simulink model "UUV_model_sim"  (R2020a)
settings: Solver=VariableStepAuto  StartTime=0.0  StopTime=20  FixedStep=0.01  RelTol=1e-3
model workspace (MAT data in the model file):
  NED = [0; 0; 0; 0; 0; 0]
  NED_dot = [0; 0; 0; 0; 0; 0]
  a = [0; 0; 0; 0; 0; 0]
  vel = [0; 0; 0; 0; 0; 0]
libraries: simulink x2
settings Model: Creator=Sebas  LastModifiedBy=Sebas

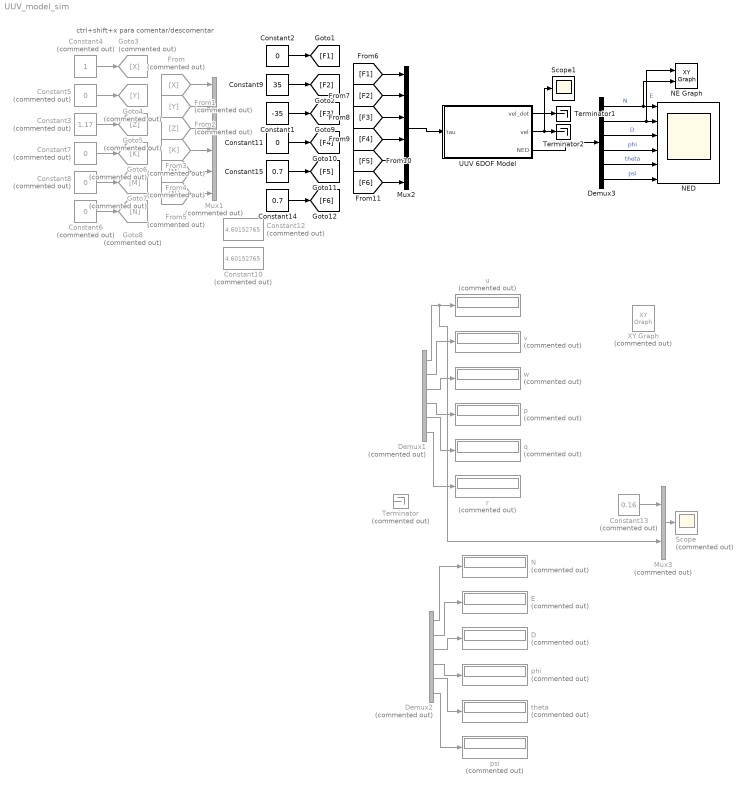
== system UUV_model_sim ==
  note: ctrl+shift+x para comentar/descomentar
  Constant1 : Constant  Value=-35
  Constant10 : Constant  Commented=on  Value=4.60152765
  Constant11 : Constant  Value=0
  Constant12 : Constant  Commented=on  Value=4.60152765
  Constant13 : Constant  Commented=on  Value=0.16
  Constant14 : Constant  Value=0.7
  Constant15 : Constant  Value=0.7
  Constant2 : Constant  Value=0
  Constant3 : Constant  Commented=on  Value=1.17
  Constant4 : Constant  Commented=on
  Constant{5..8} (4 alike) : Constant  Commented=on  Value=0
  Constant9 : Constant  Value=35
  D : Display  Commented=on
  Demux1 : Demux  Commented=on  Outputs=6
  Demux2 : Demux  Commented=on  Outputs=6
  Demux3 : Demux  Outputs=6
  E : Display  Commented=on
  From : From  Commented=on  GotoTag=X
  From1 : From  Commented=on  GotoTag=Y
  From2 : From  Commented=on  GotoTag=Z
  From3 : From  Commented=on  GotoTag=K
  From4 : From  Commented=on  GotoTag=M
  From5 : From  Commented=on  GotoTag=N
  Goto3 : Goto  Commented=on  GotoTag=X
  Goto4 : Goto  Commented=on  GotoTag=Y
  Goto5 : Goto  Commented=on  GotoTag=Z
  Goto6 : Goto  Commented=on  GotoTag=K
  Goto7 : Goto  Commented=on  GotoTag=M
  Goto8 : Goto  Commented=on  GotoTag=N
  Mux1 : Mux  Commented=on  Inputs=6
  Mux2 : Mux  Inputs=6
  Mux3 : Mux  Commented=on  Inputs=2
  N : Display  Commented=on
  NE Graph : simulink/Sinks/XY Graph  xmin=-1  xmax=5  ymin=-1  ymax=2  st=-1
  NED : Scope  NumInputPorts=6
  Scope : Scope  Commented=on
  Scope1 : Scope
  Terminator : Terminator  Commented=on
  Terminator1 : Terminator
  Terminator2 : Terminator
  UUV 6DOF Model : Subsystem
  XY Graph : simulink/Sinks/XY Graph  Commented=on  xmin=-1  xmax=1  ymin=-1  ymax=1  st=-1
  p : Display  Commented=on
  phi : Display  Commented=on
  psi : Display  Commented=on
  q : Display  Commented=on
  r : Display  Commented=on
  theta : Display  Commented=on
  u : Display  Commented=on
  v : Display  Commented=on
  w : Display  Commented=on
  wires:
  Constant4/1 -> Goto3/1
  Constant5/1 -> Goto4/1
  Constant3/1 -> Goto5/1
  Constant6/1 -> Goto8/1
  Constant8/1 -> Goto7/1
  Constant7/1 -> Goto6/1
  From1/1 -> Mux1/2
  From/1 -> Mux1/1
  From2/1 -> Mux1/3
  From4/1 -> Mux1/5
  From3/1 -> Mux1/4
  From5/1 -> Mux1/6
  Demux1/4 -> p/1
  Demux1/1 -> Mux3/2, u/1
  Demux1/5 -> q/1
  Demux1/3 -> w/1
  Demux1/2 -> v/1
  Demux1/6 -> r/1
  Demux2/5 -> theta/1
  Demux2/6 -> psi/1
  Demux2/3 -> D/1
  Demux2/2 -> E/1
  Demux2/4 -> phi/1
  Demux2/1 -> N/1
  Constant14/1 -> [F6]
  [F3] -> Mux2/3
  Constant1/1 -> [F3]
  Constant9/1 -> [F2]
  Constant2/1 -> [F1]
  [F1] -> Mux2/1
  [F4] -> Mux2/4
  [F6] -> Mux2/6
  [F5] -> Mux2/5
  Constant11/1 -> [F4]
  Constant15/1 -> [F5]
  [F2] -> Mux2/2
  Mux2/1 -> UUV 6DOF Model/1(tau)
  Mux3/1 -> Scope/1
  Constant13/1 -> Mux3/1
  UUV 6DOF Model/1(vel_dot) -> Terminator1/1
  Demux3/2 -> NE Graph/1, NED/2  "E"
  Demux3/1 -> NE Graph/2, NED/1  "N"
  UUV 6DOF Model/2(vel) -> Scope1/1, Terminator2/1
  UUV 6DOF Model/3(NED) -> Demux3/1
  Demux3/6 -> NED/6  "psi"
  Demux3/3 -> NED/3  "D"
  Demux3/4 -> NED/4  "phi"
  Demux3/5 -> NED/5  "theta"

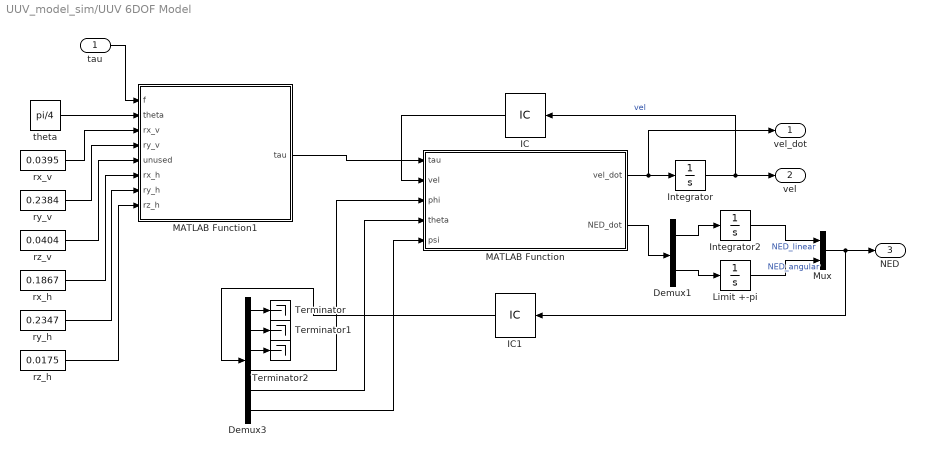
== system UUV_model_sim/UUV 6DOF Model ==
  tau : Inport
  Demux1 : Demux  Outputs=2
  Demux3 : Demux  Outputs=6
  IC : InitialCondition  Value=[0;0;0;0;0;0]
  IC1 : InitialCondition  Value=[0;0;0;0;0;0]
  Integrator : Integrator
  Integrator2 : Integrator
  Limit +-pi : Integrator  WrapState=on
  MATLAB Function : MATLAB Function  TreatAsAtomicUnit=on
  MATLAB Function1 : MATLAB Function  TreatAsAtomicUnit=on
  Mux : Mux  Inputs=2
  Terminator : Terminator
  Terminator1 : Terminator
  Terminator2 : Terminator
  rx_h : Constant  Value=0.1867
  rx_v : Constant  Value=0.0395
  ry_h : Constant  Value=0.2347
  ry_v : Constant  Value=0.2384
  rz_h : Constant  Value=0.0175
  rz_v : Constant  Value=0.0404
  theta : Constant  Value=pi/4
  vel_dot : Outport
  vel : Outport  Port=2
  NED : Outport  Port=3
  wires:
  MATLAB Function/1(vel_dot) -> vel_dot/1, Integrator/1
  Demux3/4 -> MATLAB Function/3(phi)
  Demux3/5 -> MATLAB Function/4(theta)
  Integrator/1 -> IC/1, vel/1  "vel"
  Demux3/6 -> MATLAB Function/5(psi)
  IC/1 -> MATLAB Function/2(vel)
  IC1/1 -> Demux3/1
  Demux3/2 -> Terminator1/1
  Demux3/1 -> Terminator/1
  Demux3/3 -> Terminator2/1
  MATLAB Function1/1(tau) -> MATLAB Function/1(tau)
  tau/1 -> MATLAB Function1/1(f)
  theta/1 -> MATLAB Function1/2(theta)
  rx_v/1 -> MATLAB Function1/3(rx_v)
  ry_v/1 -> MATLAB Function1/4(ry_v)
  rz_v/1 -> MATLAB Function1/5(unused)
  rx_h/1 -> MATLAB Function1/6(rx_h)
  ry_h/1 -> MATLAB Function1/7(ry_h)
  rz_h/1 -> MATLAB Function1/8(rz_h)
  Integrator2/1 -> Mux/1  "NED_linear"
  Demux1/2 -> Limit +-pi/1
  Demux1/1 -> Integrator2/1
  Mux/1 -> IC1/1, NED/1
  MATLAB Function/2(NED_dot) -> Demux1/1
  Limit +-pi/1 -> Mux/2  "NED_angular"

== matlab function UUV_model_sim/UUV 6DOF Model/MATLAB Function1 ==
  data: tau output; f input; theta input; rx_v input; ry_v input; unused input; rx_h input; ry_h input; rz_h input
function tau = tau_conversion(f, theta, rx_v, ry_v, ~, rx_h, ry_h, rz_h)
tau = [0 0 0 0 0 0].';
tau(1) = (f(1)+f(2)-f(3)-f(4))*cos(theta);
tau(2) = (-f(1)+f(2)-f(3)+f(4))*sin(theta);
tau(3) = -(f(5)+f(6));
tau(4) = (f(6)-f(5))*ry_v + (-f(1)+f(2)-f(3)+f(4))*sin(theta)*rz_h;
tau(5) = (f(6)-f(5))*rx_v + (-f(1)-f(2)+f(3)+f(4))*cos(theta)*rz_h;
tau(6) = (-f(1)+f(2)+f(3)-f(4))*(rx_h*sin(theta)+ry_h*cos(theta));

== matlab function UUV_model_sim/UUV 6DOF Model/MATLAB Function ==
  data: vel_dot output; tau input; vel input; phi input; theta input; NED_dot output; psi input
function [vel_dot,NED_dot]= UUV_forward_dynamics(tau,vel,phi,theta,psi)
% Skew symmetric matrix
S = @(s) [0    -s(3) s(2);
          s(3) 0     -s(1);
          -s(2) s(1)  0    ];  

% Vehicle parameters
m = 24;
vol = 0.02306187;
W = m*9.81;
B = W*1.005; %1000*9.81*vol;

r_g = [0 0 0].';    % Distance from origin to center of mass
r_b = [0 0 -0.10726].';    % Distance from origin to center of buoyancy
I_g = [0.900121387  -0.000186482 0.0072251;
       -0.000186482 1.754494427  0.020319615;
       0.0072251    0.020319615  1.43389     ]; % Rigid-body inertia matrix

% Rigid-Body Inertia Matrix
M_rb = [ m*eye(3)    -m*S(r_g);
         m*S(r_g)         I_g ];

% Added mass matrix
M_a = diag([16.8374 20.2748 35.3180 0.2165 0.6869 0.6157]);

% Mass matrix
M = M_rb + M_a;

% Linear damping coefficients
X_u = -0.3431;
Y_v = 0.0518;
Z_w = -0.5841;
K_p = 0.0064;
M_q = 0.04;
N_r = -0.1063;

D_lin = -diag([X_u Y_v Z_w K_p M_q N_r]);

% Cuadratic damping coefficients
X_uu = -111.7397;
Y_vv = -44.4058;
Z_ww = -157.1951;
K_pp = -0.4634;
M_qq = -0.2902;
N_rr = -2.2897;

%------------ UUV dynamic model parametrization ----------------%
% Rigid-body Coriolis-centripetal Matrix
C_rb = [ zeros(3)             -m*S(vel(1:3))-m*S(vel(4:6))*S(r_g);
        -m*S(vel(1:3))+m*S(r_g)*S(vel(4:6))            -S(I_g*vel(4:6))];

% Coreolis added mass matrix 
C_a = [ 0 0 0   0 -M_a(3,3)*vel(3) M_a(2,2)*vel(2) ;
        0 0 0   M_a(3,3)*vel(3) 0 -M_a(1,1)*vel(1) ;
        0 0 0  -M_a(2,2)*vel(2) M_a(1,1)*vel(1) 0  ;
        0 -M_a(3,3)*vel(3) M_a(2,2)*vel(2)  0 -M_a(6,6)*vel(6) M_a(5,5)*vel(5) ;
        M_a(3,3)*vel(3) 0 -M_a(1,1)*vel(1)  M_a(6,6)*vel(6) 0 -M_a(4,4)*vel(4) ;
       -M_a(2,2)*vel(2) M_a(1,1)*vel(1) 0   -M_a(5,5)*vel(5) M_a(4,4)*vel(4) 0  ];

% Coreolis matrix
C = C_rb + C_a;

% Restoring forces
g_eta = [ (W-B)*sin(theta);
          -(W-B)*cos(theta)*sin(phi);
          -(W-B)*cos(theta)*cos(phi);
          -(r_g(2)*W-r_b(2)*B)*cos(theta)*cos(phi) + (r_g(3)*W-r_b(3)*B)*cos(theta)*sin(phi);
           (r_g(3)*W-r_b(3)*B)*sin(theta)             + (r_g(1)*W-r_b(1)*B)*cos(theta)*cos(phi)
          -(r_g(1)*W-r_b(1)*B)*cos(theta)*sin(phi) - (r_g(2)*W-r_b(2)*B)*sin(theta)          ];

% Cuadratic Damping matrix
D_cuad = -diag([X_uu*abs(vel(1)) Y_vv*abs(vel(2)) Z_ww*abs(vel(3)) ...
               K_pp*abs(vel(4)) M_qq*abs(vel(5)) N_rr*abs(vel(6))]);

%Damping matrix
Damp = D_lin + D_cuad;

NED_dot = [0;0;0;0;0;0];
% Linear velocities in NED / For a zxy rotation sequence
NED_dot(1) = vel(1)*cos(psi)*cos(theta) + vel(2)*[cos(psi)*sin(theta)*sin(phi)... 
    - sin(psi)*cos(phi)] + vel(3)*[sin(psi)*sin(phi)... 
    + cos(psi)*cos(phi)*sin(theta)];

NED_dot(2) = vel(1)*sin(psi)*cos(theta) + vel(2)*[cos(psi)*cos(phi)... 
    + sin(phi)*sin(theta)*sin(psi)]+ vel(3)*[sin(theta)*sin(psi)*cos(phi)... 
    - cos(psi)*sin(phi)];

NED_dot(3) = -vel(1)*sin(theta) + vel(2)*cos(theta)*sin(phi) + vel(3)*cos(theta)*cos(phi);

%Angular velocities in NED
NED_dot(4) = vel(4) + vel(5)*sin(phi)*tan(theta) + vel(6)*cos(phi)*tan(theta);

NED_dot(5) = vel(5)*cos(phi) - vel(6)*sin(phi);

NED_dot(6) = vel(5)*(sin(phi)/cos(theta)) + vel(6)*(cos(phi)/cos(theta));

vel_dot = M\(tau-(C*vel)-(Damp*vel)-g_eta);
